simulink model "sevietta_devel_2017h"  (R2013a)
settings: Solver=VariableStepDiscrete  SolverMode=SingleTasking  StartTime=0.0  StopTime=3276  RelTol=1e-3
undefined symbols (not defined in the file): sfp
libraries: xbsIndex_r4 x2565, casper_library_delays x32, simulink x19, casper_library_misc x17, xps_library x13
(part 4 of 31)

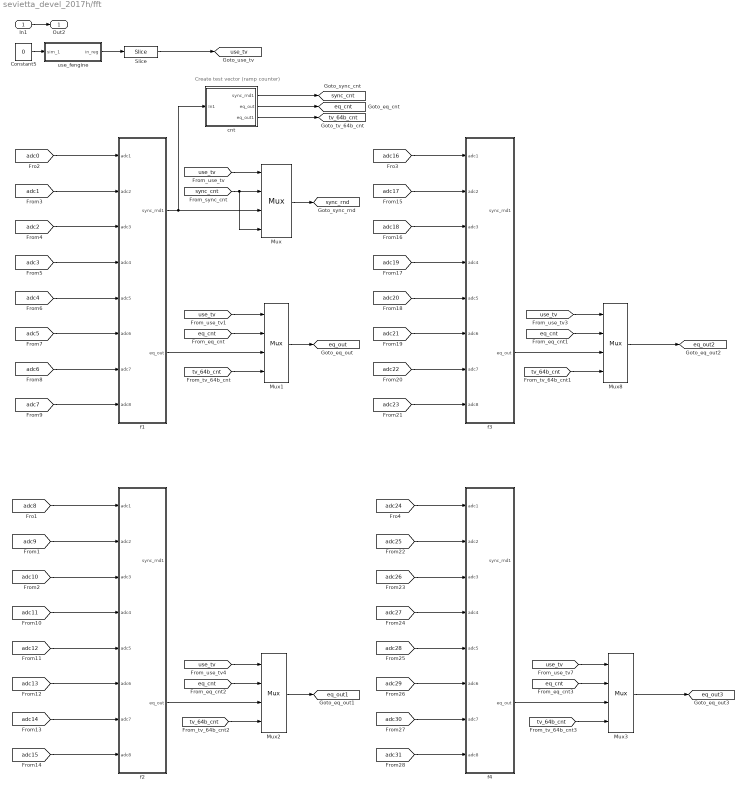
== system sevietta_devel_2017h/fft ==
  note: Create test vector (ramp counter)
  In1 : Inport
  Constant5 : Constant  Value=0  SampleTime=1/4
  Mux{,1..3,8} (5 alike) : xbsIndex_r4/Mux  inputs=3  en=off  latency=1  precision=Full  arith_type=Unsigned  n_bits=16  bin_pt=14  quantization=Truncate  overflow=Wrap  dbl_ovrd=off  block_type=mux
  Slice : xbsIndex_r4/Slice  nbits=2  boolean_output=off  mode=Lower Bit Location + Width  bit1=0  base1=MSB of Input  bit0=0  base0=LSB of Input  dbl_ovrd=off  block_type=slice
  cnt : Subsystem
  f1 : Subsystem
  f2 : Subsystem
  f3 : Subsystem
  f4 : Subsystem
  use_fengine : Subsystem  Tag=xps:sw_reg  AncestorBlock=xps_library/software_register  mask(swreg){mode=one value, io_dir=From Processor, io_delay=0, sample_period=1, names=reg, bitwidths=32, arith_types=0, bin_pts=0, sim_port=on, show_format=off}
      mask prompts: io_dir "I/O direction"; io_delay "I/O delay"; sample_period "Sample period"; names "Name:"; bitwidths "Bitwidth:"; arith_types "Type (ufix=0, fix=1, bool=2):"; bin_pts "Binary pt:"; sim_port "Provide sim input/output?"; show_format "Print format string?"
      mask init:
      | swreg_init(gcb)
      settings: AttributesFormatString=1input
      mask TypeOptions mode: one value | fields of equal size | fields of arbitrary size
      mask Callback mode: swreg_cb(gcb);
      mask TypeOptions io_dir: To Processor | From Processor
      mask Callback io_dir:
      | mask_enables = get_param(gcb, 'MaskEnables');
      | mask_names = get_param(gcb, 'MaskNames');
      | if strcmp(get_param(gcb, 'io_dir'), 'To Processor'),
      |     mask_enables{ismember(mask_names, 'sample_period')} = 'off';
      | else
      |     mask_enables{ismember(mask_names, 'sample_period')} = 'on';
      | end
      | set_param(gcb, 'MaskEnables', mask_enables);
      mask Callback bitwidths:
      | swreg_maskcheck(gcb);
      | % blk = gcb;
      | % mode = get_param(blk, 'mode');
      | % current_widths = eval(get_param(blk, 'bitwidths'));
      | % if (strcmp(mode, 'one value') || strcmp(mode, 'fields of equal size')) && (length(current_widths) > 1),
      | %     error('Only one width may be specified for this mode.');
      | % elseif strcmp(mode, 'fields of arbitrary size')
      | %     current_names = textscan(strtrim(strrep(strrep(get_param(blk, 'names'), ']', ''), '[', '')), '%s');
      | %     current_names = current_names{1};
      | %     numios = length(current_names);
      | %     if length(current_widths) ~= numios,
      | %         error('%d field names specified, but %d widths?', numios, length(current_widths));
      | %     end
      | % end
      | % total_width = 0;
      | % for ctr = 1 : length(current_widths),
      | %     total_width = total_width + current_widths(ctr);
      | % end
      | % if total_width > 32,
      | %     error('Total width must be 32 or less, set to %d.', total_width);
      | % end
      mask Callback arith_types:
      | [numios, ~, ~, ~, current_types] = swreg_maskcheck(gcb);
      | % blk = gcb;
      | % mode = get_param(blk, 'mode');
      | % current_types = eval(get_param(blk, 'arith_types'));
      | % numios = length(current_types);
      | % if (strcmp(mode, 'one value') || strcmp(mode, 'fields of equal size')) && (length(current_types) > 1),
      | %     error('Only one type may be specified for this mode.');
      | % elseif strcmp(mode, 'fields of arbitrary size')
      | %     current_names = textscan(strtrim(strrep(strrep(get_param(blk, 'names'), ']', ''), '[', '')), '%s');
      | %     current_names = current_names{1};
      | %     numios = length(current_names);
      | %     if length(current_types) ~= numios,
      | %         error('%d field names specified, but %d types?', numios, length(current_types));
      | %     end
      | % end
      | problem = 0;
      | for ctr = 1 : numios,
      |     t = current_types(ctr);
      |     if (t < 0) || (t > 2),
      |         problem = t;
      |         ctr = numios + 1;
      |     end
      | end
      | if problem ~= 0,
      |     error('Type cannot be %i, must be 0, 1 or 2.', problem);
      | end
      mask Callback bin_pts:
      | swreg_maskcheck(gcb);
      | % blk = gcb;
      | % mode = get_param(blk, 'mode');
      | % current_bins = eval(get_param(blk, 'bin_pts'));
      | % if (strcmp(mode, 'one value') || strcmp(mode, 'fields of equal size')) && (length(current_bins) > 1),
      | %     error('Only one binary pt may be specified for this mode.');
      | % elseif strcmp(mode, 'fields of arbitrary size')
      | %     current_names = textscan(strtrim(strrep(strrep(get_param(blk, 'names'), ']', ''), '[', '')), '%s');
      | %     current_names = current_names{1};
      | %     numios = length(current_names);
      | %     if length(current_bins) ~= numios,
      | %         error('%d field names specified, but %d binary pts?', numios, length(current_bins));
      | %     end
      | % end
  Out2 : Outport
  tag scope: eq_cnt=global, eq_out1=global, eq_out2=global, eq_out3=global, eq_out=global, sync_cnt=global, sync_rnd=global, tv_64b_cnt=global, use_tv=global
  wires:
  In1/1 -> Out2/1
  [adc0] -> f1/1(adc1)
  [adc1] -> f1/2(adc2)
  [adc2] -> f1/3(adc3)
  [adc3] -> f1/4(adc4)
  [adc4] -> f1/5(adc5)
  [adc5] -> f1/6(adc6)
  [adc6] -> f1/7(adc7)
  [adc7] -> f1/8(adc8)
  [adc10] -> f2/3(adc3)
  [adc14] -> f2/7(adc7)
  [adc11] -> f2/4(adc4)
  [adc12] -> f2/5(adc5)
  [adc13] -> f2/6(adc6)
  [adc8] -> f2/1(adc1)
  [adc15] -> f2/8(adc8)
  [adc9] -> f2/2(adc2)
  [adc21] -> f3/6(adc6)
  [adc22] -> f3/7(adc7)
  [adc23] -> f3/8(adc8)
  [adc18] -> f3/3(adc3)
  [adc19] -> f3/4(adc4)
  [adc20] -> f3/5(adc5)
  [adc17] -> f3/2(adc2)
  [adc16] -> f3/1(adc1)
  [adc25] -> f4/2(adc2)
  [adc24] -> f4/1(adc1)
  [adc29] -> f4/6(adc6)
  [adc26] -> f4/3(adc3)
  [adc27] -> f4/4(adc4)
  [adc28] -> f4/5(adc5)
  [adc30] -> f4/7(adc7)
  [adc31] -> f4/8(adc8)
  use_fengine/1(in_reg) -> Slice/1
  Constant5/1 -> use_fengine/1(sim_1)
  cnt/1(sync_rnd1) -> [sync_cnt]
  cnt/2(eq_out) -> [eq_cnt]
  [use_tv] -> Mux/1
  f1/1(sync_rnd1) -> cnt/1(In1), Mux/3
  [sync_cnt] -> Mux/4, Mux/2
  Mux/1 -> [sync_rnd]
  [use_tv] -> Mux1/1
  Mux1/1 -> [eq_out]
  [eq_cnt] -> Mux1/2
  [use_tv] -> Mux8/1
  [eq_cnt] -> Mux8/2
  Mux8/1 -> [eq_out2]
  [use_tv] -> Mux2/1
  [eq_cnt] -> Mux2/2
  Mux2/1 -> [eq_out1]
  [use_tv] -> Mux3/1
  [eq_cnt] -> Mux3/2
  Mux3/1 -> [eq_out3]
  f1/2(eq_out) -> Mux1/3
  f2/2(eq_out) -> Mux2/3
  f4/2(eq_out) -> Mux3/3
  f3/2(eq_out) -> Mux8/3
  Slice/1 -> [use_tv]
  cnt/3(eq_out1) -> [tv_64b_cnt]
  [tv_64b_cnt] -> Mux1/4
  [tv_64b_cnt] -> Mux8/4
  [tv_64b_cnt] -> Mux2/4
  [tv_64b_cnt] -> Mux3/4
